simulink model "model_biquad"  (R2020b)
settings: Solver=VariableStepAuto  StartTime=0.0  StopTime=32e-3  RelTol=1e-3
values from neighbouring files (symbols this model uses):
  in_cos = 2*cos(2*pi*k/N)    [compute_constants.m]    (also in signat_to_test_generate.m = -2*cos(2*pi*k/N))
  Ts = 1e-3    (= 0.001)    [compute_constants.m]    (also in signat_to_test_generate.m)
  Wkn = -exp(-j*2*pi*k/N)    [compute_constants.m]    (also in signat_to_test_generate.m)
undefined symbols (not defined in the file or in its folder): dfilt
libraries: dsparch4 x1
settings Model: Creator=pablo  LastModifiedBy=pablo

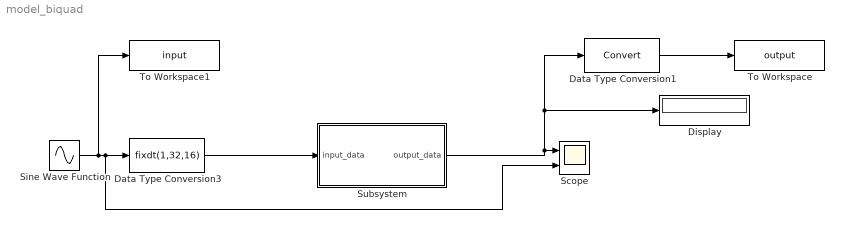
== system model_biquad ==
  Data Type Conversion1 : DataTypeConversion
  Data Type Conversion3 : DataTypeConversion  OutDataTypeStr=fixdt(1,32,16)
  Display : Display
  Scope : Scope  NumInputPorts=2
  Sine Wave Function : Sin  SineType=Sample based  Samples=32  SampleTime=Ts  Offset=4
  Subsystem : Subsystem
  To Workspace : ToWorkspace  VariableName=output  SampleTime=Ts
  To Workspace1 : ToWorkspace  VariableName=input  SampleTime=Ts
  wires:
  Subsystem/1(output_data) -> Display/1, Data Type Conversion1/1, Scope/1
  Data Type Conversion1/1 -> To Workspace/1
  Data Type Conversion3/1 -> Subsystem/1(input_data)
  Sine Wave Function/1 -> To Workspace1/1, Scope/2, Data Type Conversion3/1

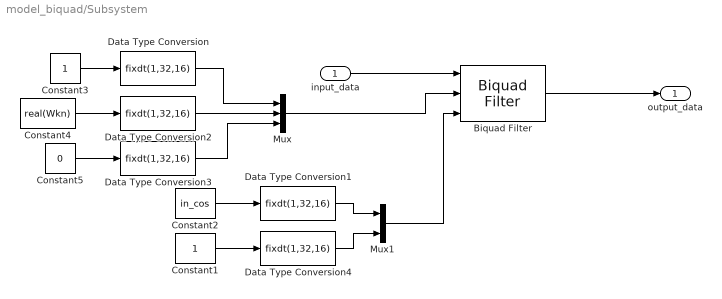
== system model_biquad/Subsystem ==
  input_data : Inport  OutDataTypeStr=fixdt(1,32,16)  SampleTime=Ts
  Biquad Filter : dsparch4/Biquad Filter  FilterSource=Input port(s)  CoeffSource=Specify via dialog  FilterObject=dfilt.df2tsos([1 0.3 0.4],[1 0.1 0.2])  IIRFiltStruct=Direct form II transposed  BiQuadCoeffs=[0 1 real(Wkn) 1 -in_cos 1]  ScaleValues=1  IC=0  ICnum=0  ICden=0  a0Flag=Warning  optimizeScaleValues=on  ScaleValueMode=Assume all are unity and optimize  roundingMode=Floor  overflowMode=off  scaleValueFracLength=14  denProdOutputFracLength=30  denAccumFracLength=30  secondMemoryFracLength=15
      settings: SourceProductName=DSP System Toolbox
  Constant1 : Constant
  Constant2 : Constant  Value=in_cos
  Constant3 : Constant
  Constant4 : Constant  Value=real(Wkn)
  Constant5 : Constant  Value=0
  Data Type Conversion{,1..4} (5 alike) : DataTypeConversion  OutDataTypeStr=fixdt(1,32,16)
  Mux : Mux  Inputs=3
  Mux1 : Mux  Inputs=2
  output_data : Outport  InitialOutput=0
  wires:
  Constant5/1 -> Data Type Conversion3/1
  Biquad Filter/1 -> output_data/1
  input_data/1 -> Biquad Filter/1
  Constant3/1 -> Data Type Conversion/1
  Constant2/1 -> Data Type Conversion1/1
  Constant1/1 -> Data Type Conversion4/1
  Mux/1 -> Biquad Filter/2
  Mux1/1 -> Biquad Filter/3
  Data Type Conversion/1 -> Mux/1
  Constant4/1 -> Data Type Conversion2/1
  Data Type Conversion2/1 -> Mux/2
  Data Type Conversion3/1 -> Mux/3
  Data Type Conversion1/1 -> Mux1/1
  Data Type Conversion4/1 -> Mux1/2
